simulink model "odev2_iremelmas_kara"  (R2023b)
settings: Solver=ode23tb  StartTime=0.0  StopTime=3  MaxStep=1e-5  RelTol=1e-3
undefined symbols (not defined in the file or in its folder): DiscIntNeverNeededParam
libraries: spsSeriesRLCBranchLib x5, spsDiodeLib x1, spsDCVoltageSourceLib x1, spsGroundLib x1, spsIGBTLib x1, SignalEditorBlockLib x1, spsVoltageMeasurementLib x1, sps_lib x1
settings Model: Creator=ireme  LastModifiedBy=ireme

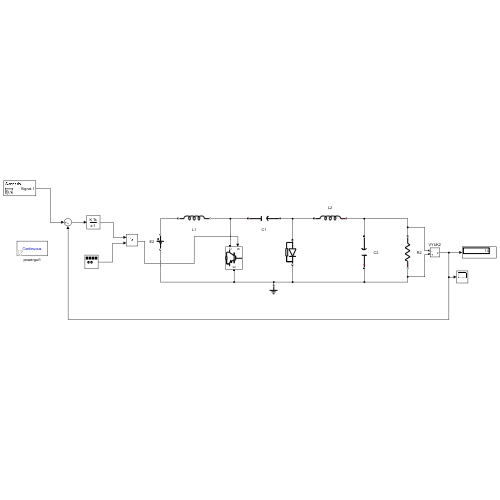
[thumbnail: Simulink's stored preview of the top-level diagram]
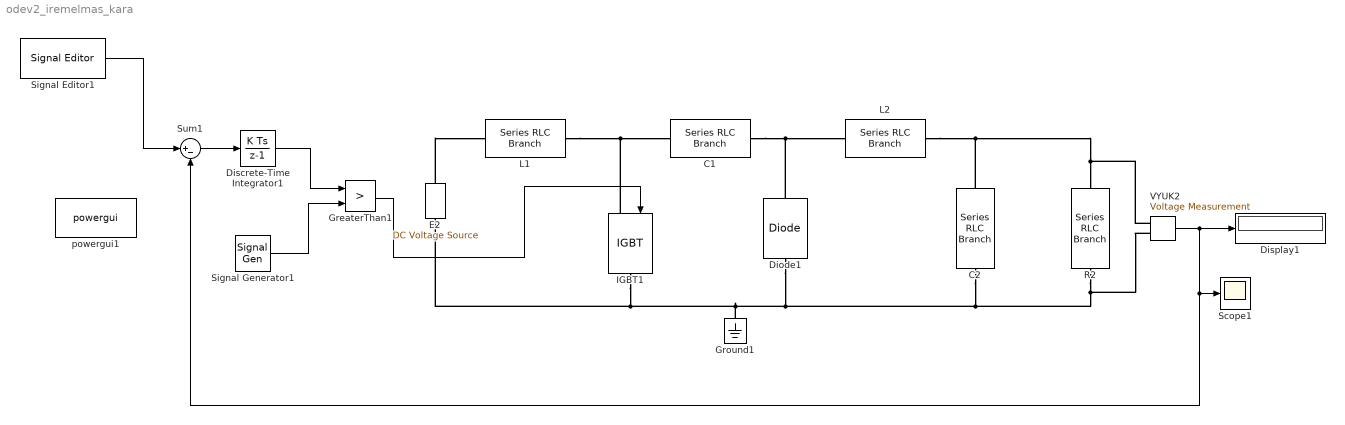
== system odev2_iremelmas_kara ==
  C1 : spsSeriesRLCBranchLib/Series RLC Branch  LConnTagsString=__new0  RConnTagsString=__new0  BranchType=C  Resistance=1  Inductance=180e-6  SetiL0=off  InitialCurrent=0  Capacitance=200e-6  Setx0=off  InitialVoltage=0  Measurements=None
  C2 : spsSeriesRLCBranchLib/Series RLC Branch  LConnTagsString=__new0  RConnTagsString=__new0  BranchType=C  Resistance=1  Inductance=180e-6  SetiL0=off  InitialCurrent=0  Capacitance=220e-6  Setx0=off  InitialVoltage=0  Measurements=None
  Diode1 : spsDiodeLib/Diode  Ron=0.0001  Lon=0  Vf=0.001  IC=0  UseSnubber=0  Rs=5000  Cs=250e-6  Measurements=off
  Discrete-Time Integrator1 : DiscreteIntegrator  gainval=10  SampleTime=3e-6  ICPrevOutput=DiscIntNeverNeededParam  ICPrevScaledInput=DiscIntNeverNeededParam
  Display1 : Display
  E2 : spsDCVoltageSourceLib/DC Voltage Source  Amplitude=12  Measurements=None
  GreaterThan1 : RelationalOperator  Operator=>  OutDataTypeStr=boolean  RndMeth=Simplest  InputSameDT=off
  Ground1 : spsGroundLib/Ground  LConnTagsString=a
  IGBT1 : spsIGBTLib/IGBT  Ron=0.000001  Lon=0  Vf=0.00001  Tf=1e-6  Tt=2e-6  IC=0  Rs=1e5  Cs=inf  Measurements=off
  L1 : spsSeriesRLCBranchLib/Series RLC Branch  LConnTagsString=__new0  RConnTagsString=__new0  BranchType=L  Resistance=1  Inductance=180e-6  SetiL0=off  InitialCurrent=0  Capacitance=1e-6  Setx0=off  InitialVoltage=0  Measurements=None
  L2 : spsSeriesRLCBranchLib/Series RLC Branch  LConnTagsString=__new0  RConnTagsString=__new0  BranchType=L  Resistance=1  Inductance=150e-6  SetiL0=off  InitialCurrent=0  Capacitance=1e-6  Setx0=off  InitialVoltage=0  Measurements=None
  R2 : spsSeriesRLCBranchLib/Series RLC Branch  LConnTagsString=__new0  RConnTagsString=__new0  BranchType=R  Resistance=3.2  Inductance=180e-6  SetiL0=off  InitialCurrent=0  Capacitance=1e-6  Setx0=off  InitialVoltage=0  Measurements=None
  Scope1 : Scope
  Signal Generator1 : SignalGenerator  WaveForm=sawtooth  Frequency=25e3
  Signal Editor1 : SignalEditorBlockLib/Signal Editor  FileName=D:\simulink_odev\odev2_iremelmas_kara\odev2_iremelmas_kara.mat  ActiveScenario=Scenario  ActiveSignal=Signal 1  IsBus=off  OutputBusObjectStr=Bus: BusObject  SampleTime=0  Interpolate=off  ZeroCross=off  OutputAfterFinalValue=Setting to zero  Unit=inherit  PreserveSignalName=on  ApplySigPropsToAllScenarios=on  ApplySigPropsToAllSignals=off
  Sum1 : Sum  Inputs=|+-
  VYUK2 : spsVoltageMeasurementLib/Voltage Measurement  PhasorSimulation=off  OutputType=Complex  PSBequivalent=0
  powergui1 : sps_lib/powergui  Priority=1  SimulationMode=Continuous  SampleTime=50e-6  frequency=60  Iterations=50  frequencyindice=0  Pbase=100e6  ErrMax=1e-4  UnitsV=kV  UnitsW=MW  buscounter=0  FunctionMessages=off  echomessages=off  EnableUseOfTLC=off  CurrentSourceSwitches=off  DisableSnubberDevices=off  DisableRonSwitches=off  DisableVfSwitches=off  DisplayEquations=off  AutomaticDiscreteSolvers=off  SolverType=Tustin/Backward Euler (TBE)  Interpol=off  ExternalGateDelay=off  methode=off  Ts=100  x0status=blocks  SPID=on  SwTol=0  HookPort=off  NonlinearTolerance=1e-4  nMaxIteration=100  ContinueOnMaxIteration=off  RestoreLinks=warning  ResistiveCurrentMeasurement=off  Frange=[0:2:500]  Ylog=off  Xlog=on  ShowGrid=off  save=off  variable=ZData  structure=0  ZoomFFT=off  StartTime=0.0  cycles=1  DisplayStyle=1  fundamental=60  FreqAxis=off  MaxFrequency=1000  frequencyindicesteady=1  RmsSteady=1  display=off
  wires:
  Signal Editor1/1 -> Sum1/1
  GreaterThan1/1 -> IGBT1/1
  VYUK2/1 -> Display1/1, Scope1/1, Sum1/2
  Discrete-Time Integrator1/1 -> GreaterThan1/1
  Signal Generator1/1 -> GreaterThan1/2
  Sum1/1 -> Discrete-Time Integrator1/1
  connections:
  R2/LConn1 -- VYUK2/LConn1 -- C2/LConn1 -- Diode1/RConn1 -- Ground1/LConn1 -- IGBT1/RConn1 -- E2/LConn1
  L1/RConn1 -- IGBT1/LConn1 -- C1/LConn1
  C2/RConn1 -- VYUK2/LConn2 -- R2/RConn1 -- L2/LConn1
  C1/RConn1 -- Diode1/LConn1 -- L2/RConn1
  E2/RConn1 -- L1/LConn1
